simulink model "Electron_Energization_new_test"  (R2020a)
settings: Solver=ode45  StartTime=0.0  StopTime=t_stamp(end)  RelTol=1e-3  EnableMultiTasking=on
values from neighbouring files (symbols this model uses):
  E0 = 1e6    (= 1000000)    [windmi.m]
  Gain_factor_I1 = 1    [test_2taus.m]    (also in windmi.m)
  t_delay_E_index = 10    [test_2taus.m]    (also in windmi.m = 0)
  tau_loss1 = 100    [test_2taus.m]    (also in windmi.m = 1)
settings Model: Creator=edmund  LastModifiedBy=pavit
settings DataIOCC: SaveFormat=Array  ReturnWorkspaceOutputs=off  TimeSaveName=tout_E  OutputSaveName=yout_E
settings OptimizationCC: LifeSpan=inf
settings DebuggingCC: SFUnexpectedBacktrackingDiag=warning  SFNoUnconditionalDefaultTransitionDiag=warning  SFExecutionAtInitializationDiag=none  ArithmeticOperatorsInVariantConditions=warning
settings HardwareCC: ProdBitPerPointer=32  ProdBitPerSizeT=32  ProdBitPerPtrDiffT=32  ProdLargestAtomicFloat=None  ProdIntDivRoundTo=Undefined  ProdEndianess=Unspecified  ProdWordSize=32  ProdHWDeviceType=32-bit Generic
settings ModelReferenceCC: PropagateSignalLabelsOutOfModel=off
settings SFSimCC: SimUseLocalCustomCode=off  CustomCodeUndefinedFunction=UseInterfaceOnly
settings RTWCC: RTWUseLocalCustomCode=off
settings CodeAppCC: StateflowObjectComments=on
settings GRTTargetCC: TargetLangStandard=C89/C90 (ANSI)
settings ConfigComp: CovMetricSettings=dw  CovHtmlReporting=on  CovSaveCumulativeToWorkspaceVar=on  CovSaveSingleToWorkspaceVar=on  CovExternalEMLEnable=off  CovSFcnEnable=off

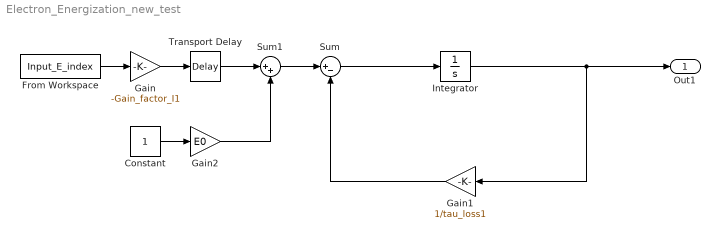
== system Electron_Energization_new_test ==
  Constant : Constant
  From Workspace : FromWorkspace  VariableName=Input_E_index
  Gain : Gain  Gain=-Gain_factor_I1
  Gain1 : Gain  Gain=1/tau_loss1
  Gain2 : Gain  Gain=E0
  Integrator : Integrator
  Sum : Sum  Inputs=|+-
  Sum1 : Sum  Inputs=|++
  Transport Delay : TransportDelay  DelayTime=t_delay_E_index
  Out1 : Outport
  wires:
  Integrator/1 -> Out1/1, Gain1/1
  Gain1/1 -> Sum/2
  From Workspace/1 -> Gain/1
  Sum/1 -> Integrator/1
  Gain/1 -> Transport Delay/1
  Transport Delay/1 -> Sum1/1
  Sum1/1 -> Sum/1
  Constant/1 -> Gain2/1
  Gain2/1 -> Sum1/2
